simulink library "twolinkslib"  (R2019a)
settings: Solver=VariableStepAuto  StartTime=0.0  StopTime=10.0  RelTol=1e-3
libraries: $bdroot x5
settings Model: Creator=ah501846  LastModifiedBy=ah501846

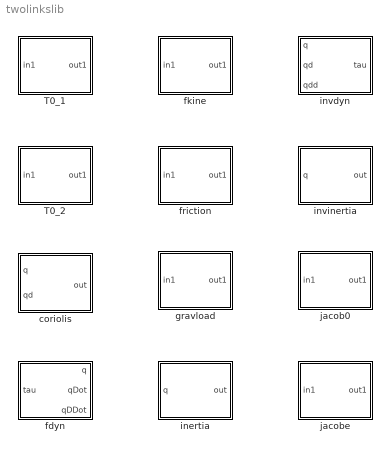
== system twolinkslib ==
  T0_1 : MATLAB Function  TreatAsAtomicUnit=on
  T0_2 : MATLAB Function  TreatAsAtomicUnit=on
  coriolis : Subsystem
  fdyn : Subsystem
  fkine : MATLAB Function  TreatAsAtomicUnit=on
  friction : MATLAB Function  TreatAsAtomicUnit=on
  gravload : MATLAB Function  TreatAsAtomicUnit=on
  inertia : Subsystem
  invdyn : Subsystem
  invinertia : Subsystem
  jacob0 : MATLAB Function  TreatAsAtomicUnit=on
  jacobe : MATLAB Function  TreatAsAtomicUnit=on

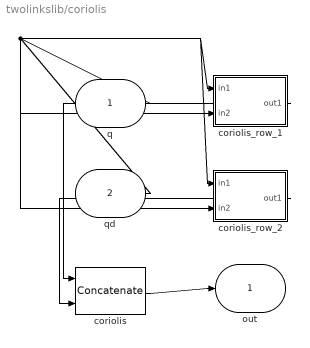
== system twolinkslib/coriolis ==
  q : Inport
  qd : Inport  Port=2
  coriolis : Concatenate  Mode=Multidimensional array
  coriolis_row_1 : MATLAB Function  TreatAsAtomicUnit=on
  coriolis_row_2 : MATLAB Function  TreatAsAtomicUnit=on
  out : Outport
  wires:
  coriolis/1 -> out/1
  coriolis_row_1/1(out1) -> coriolis/1
  q/1 -> coriolis_row_1/1(in1), coriolis_row_2/1(in1)
  qd/1 -> coriolis_row_1/2(in2), coriolis_row_2/2(in2)
  coriolis_row_2/1(out1) -> coriolis/2

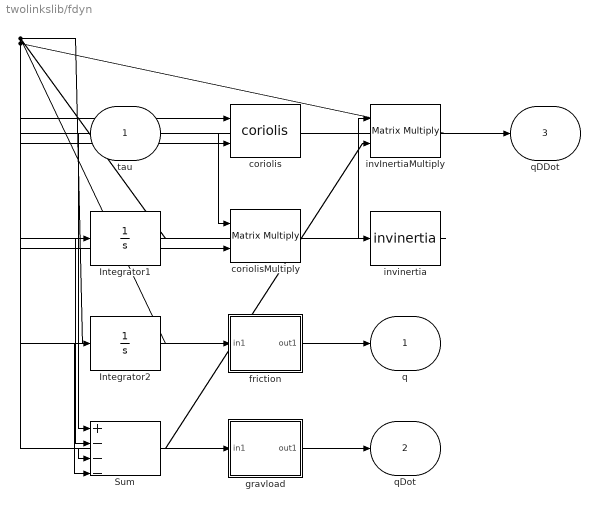
== system twolinkslib/fdyn ==
  tau : Inport
  Integrator1 : Integrator
  Integrator2 : Integrator
  Sum : Sum  Inputs=|+---  SaturateOnIntegerOverflow=on  InputSameDT=on  OutDataTypeStr=Inherit: Same as first input
  coriolis : $bdroot/coriolis  SystemSampleTime=-1
  coriolisMultiply : Product  Multiplication=Matrix(*)  SaturateOnIntegerOverflow=on  RndMeth=Zero  InputSameDT=on  OutDataTypeStr=Inherit: Same as first input
  friction : MATLAB Function  TreatAsAtomicUnit=on
  gravload : MATLAB Function  TreatAsAtomicUnit=on
  invInertiaMultiply : Product  Multiplication=Matrix(*)  SaturateOnIntegerOverflow=on  RndMeth=Zero  InputSameDT=on  OutDataTypeStr=Inherit: Same as first input
  invinertia : $bdroot/invinertia  SystemSampleTime=-1
  q : Outport
  qDot : Outport  Port=2
  qDDot : Outport  Port=3
  wires:
  tau/1 -> Sum/1
  invInertiaMultiply/1 -> qDDot/1, Integrator1/1
  Integrator1/1 -> Integrator2/1, qDot/1, coriolis/2, coriolisMultiply/2, friction/1(in1)
  Integrator2/1 -> q/1, coriolis/1, gravload/1(in1), invinertia/1
  invinertia/1 -> invInertiaMultiply/1
  Sum/1 -> invInertiaMultiply/2
  coriolisMultiply/1 -> Sum/2
  gravload/1(out1) -> Sum/3
  friction/1(out1) -> Sum/4
  coriolis/1 -> coriolisMultiply/1

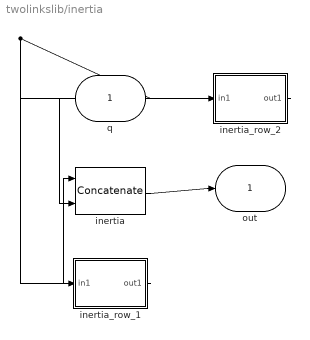
== system twolinkslib/inertia ==
  q : Inport
  inertia : Concatenate  Mode=Multidimensional array
  inertia_row_1 : MATLAB Function  TreatAsAtomicUnit=on
  inertia_row_2 : MATLAB Function  TreatAsAtomicUnit=on
  out : Outport
  wires:
  inertia/1 -> out/1
  inertia_row_1/1(out1) -> inertia/1
  q/1 -> inertia_row_1/1(in1), inertia_row_2/1(in1)
  inertia_row_2/1(out1) -> inertia/2

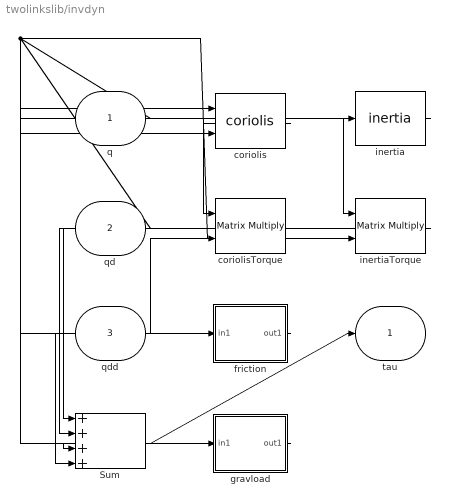
== system twolinkslib/invdyn ==
  q : Inport
  qd : Inport  Port=2
  qdd : Inport  Port=3
  Sum : Sum  Inputs=++++  SaturateOnIntegerOverflow=on  InputSameDT=on  OutDataTypeStr=Inherit: Same as first input
  coriolis : $bdroot/coriolis  SystemSampleTime=-1
  coriolisTorque : Product  Multiplication=Matrix(*)  SaturateOnIntegerOverflow=on  RndMeth=Zero  InputSameDT=on  OutDataTypeStr=Inherit: Same as first input
  friction : MATLAB Function  TreatAsAtomicUnit=on
  gravload : MATLAB Function  TreatAsAtomicUnit=on
  inertia : $bdroot/inertia  SystemSampleTime=-1
  inertiaTorque : Product  Multiplication=Matrix(*)  SaturateOnIntegerOverflow=on  RndMeth=Zero  InputSameDT=on  OutDataTypeStr=Inherit: Same as first input
  tau : Outport
  wires:
  q/1 -> inertia/1, coriolis/1, gravload/1(in1)
  qd/1 -> coriolis/2, friction/1(in1), coriolisTorque/2
  inertia/1 -> inertiaTorque/1
  qdd/1 -> inertiaTorque/2
  coriolis/1 -> coriolisTorque/1
  inertiaTorque/1 -> Sum/1
  coriolisTorque/1 -> Sum/2
  gravload/1(out1) -> Sum/3
  friction/1(out1) -> Sum/4
  Sum/1 -> tau/1

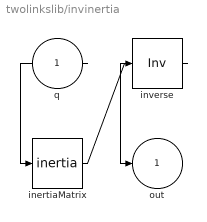
== system twolinkslib/invinertia ==
  q : Inport
  inertiaMatrix : $bdroot/inertia  SystemSampleTime=-1
  inverse : Product  Inputs=/  Multiplication=Matrix(*)
  out : Outport
  wires:
  q/1 -> inertiaMatrix/1
  inertiaMatrix/1 -> inverse/1
  inverse/1 -> out/1

== matlab function twolinkslib/inertia/inertia_row_2 ==
  data: in1 input; out1 output
function out1 = inertia_row_2(in1)
%#codegen

%    This function was generated by the Symbolic Math Toolbox version 8.3.
%    26-Apr-2019 09:45:12

q2 = in1(:,2);
out1 = [cos(q2)./2.0+1.0./4.0,1.0./4.0];

== matlab function twolinkslib/inertia/inertia_row_1 ==
  data: in1 input; out1 output
function out1 = inertia_row_1(in1)
%#codegen

%    This function was generated by the Symbolic Math Toolbox version 8.3.
%    26-Apr-2019 09:45:12

q2 = in1(:,2);
t2 = cos(q2);
out1 = [t2+3.0./2.0,t2./2.0+1.0./4.0];

== matlab function twolinkslib/fkine ==
  data: in1 input; out1 output
function out1 = fkine(in1)
%#codegen

%    This function was generated by the Symbolic Math Toolbox version 8.3.
%    26-Apr-2019 09:45:03

q1 = in1(:,1);
q2 = in1(:,2);
t2 = q1+q2;
t3 = cos(t2);
t4 = sin(t2);
out1 = reshape([t3,0.0,t4,0.0,-t4,0.0,t3,0.0,0.0,-1.0,0.0,0.0,t3+cos(q1),0.0,t4+sin(q1),1.0],[4,4]);

== matlab function twolinkslib/T0_1 ==
  data: in1 input; out1 output
function out1 = T0_1(in1)
%#codegen

%    This function was generated by the Symbolic Math Toolbox version 8.3.
%    26-Apr-2019 09:45:03

q1 = in1(:,1);
t2 = cos(q1);
t3 = sin(q1);
out1 = reshape([t2,0.0,t3,0.0,-t3,0.0,t2,0.0,0.0,-1.0,0.0,0.0,t2,0.0,t3,1.0],[4,4]);

== matlab function twolinkslib/T0_2 ==
  data: in1 input; out1 output
function out1 = T0_2(in1)
%#codegen

%    This function was generated by the Symbolic Math Toolbox version 8.3.
%    26-Apr-2019 09:45:04

q1 = in1(:,1);
q2 = in1(:,2);
t2 = cos(q1);
t3 = cos(q2);
t4 = sin(q1);
t5 = sin(q2);
t6 = t2.*t3;
t7 = t2.*t5;
t8 = t3.*t4;
t9 = t4.*t5;
t10 = -t9;
t11 = t6+t10;
out1 = reshape([t11,0.0,t7+t8,0.0,-t7-t8,0.0,t11,0.0,0.0,-1.0,0.0,0.0,t2+t11,0.0,t4+t7+t8,1.0],[4,4]);

== matlab function twolinkslib/jacob0 ==
  data: in1 input; out1 output
function out1 = jacob0(in1)
%#codegen

%    This function was generated by the Symbolic Math Toolbox version 8.3.
%    26-Apr-2019 09:45:06

q1 = in1(:,1);
q2 = in1(:,2);
t2 = cos(q2);
t3 = sin(q2);
t4 = q1+q2;
t5 = t2+1.0;
t6 = cos(t4);
t7 = sin(t4);
out1 = reshape([t3.*t6-t5.*t7,0.0,t3.*t7+t5.*t6,0.0,-1.0,0.0,-t7,0.0,t6,0.0,-1.0,0.0],[6,2]);

== matlab function twolinkslib/jacobe ==
  data: in1 input; out1 output
function out1 = jacobe(in1)
%#codegen

%    This function was generated by the Symbolic Math Toolbox version 8.3.
%    26-Apr-2019 09:45:07

q2 = in1(:,2);
out1 = reshape([sin(q2),cos(q2)+1.0,0.0,0.0,0.0,1.0,0.0,1.0,0.0,0.0,0.0,1.0],[6,2]);

== matlab function twolinkslib/gravload ==
  data: in1 input; out1 output
function out1 = gravload(in1)
%#codegen

%    This function was generated by the Symbolic Math Toolbox version 8.3.
%    26-Apr-2019 09:45:09

q1 = in1(:,1);
q2 = in1(:,2);
t2 = q1+q2;
t3 = cos(t2);
t4 = t3.*(9.81e+2./2.0e+2);
out1 = [t4+cos(q1).*1.4715e+1,t4];

== matlab function twolinkslib/coriolis/coriolis_row_1 ==
  data: in1 input; out1 output; in2 input
function out1 = coriolis_row_1(in1,in2)
%#codegen

%    This function was generated by the Symbolic Math Toolbox version 8.3.
%    26-Apr-2019 09:45:16

q2 = in1(:,2);
qd1 = in2(:,1);
qd2 = in2(:,2);
t2 = sin(q2);
out1 = [qd2.*t2.*(-1.0./2.0),t2.*(qd1+qd2).*(-1.0./2.0)];

== matlab function twolinkslib/coriolis/coriolis_row_2 ==
  data: in1 input; out1 output; in2 input
function out1 = coriolis_row_2(in1,in2)
%#codegen

%    This function was generated by the Symbolic Math Toolbox version 8.3.
%    26-Apr-2019 09:45:16

q2 = in1(:,2);
qd1 = in2(:,1);
out1 = [(qd1.*sin(q2))./2.0,0.0];

== matlab function twolinkslib/friction ==
  data: in1 input; out1 output
function out1 = friction(in1)
%#codegen

%    This function was generated by the Symbolic Math Toolbox version 8.3.
%    26-Apr-2019 09:45:18

out1 = [0.0,0.0];

== matlab function twolinkslib/fdyn/gravload ==
  data: in1 input; out1 output
function out1 = gravload(in1)
%#codegen

%    This function was generated by the Symbolic Math Toolbox version 8.3.
%    26-Apr-2019 09:45:09

q1 = in1(:,1);
q2 = in1(:,2);
t2 = q1+q2;
t3 = cos(t2);
t4 = t3.*(9.81e+2./2.0e+2);
out1 = [t4+cos(q1).*1.4715e+1,t4];

== matlab function twolinkslib/fdyn/friction ==
  data: in1 input; out1 output
function out1 = friction(in1)
%#codegen

%    This function was generated by the Symbolic Math Toolbox version 8.3.
%    26-Apr-2019 09:45:18

out1 = [0.0,0.0];

== matlab function twolinkslib/invdyn/gravload ==
  data: in1 input; out1 output
function out1 = gravload(in1)
%#codegen

%    This function was generated by the Symbolic Math Toolbox version 8.3.
%    26-Apr-2019 09:45:09

q1 = in1(:,1);
q2 = in1(:,2);
t2 = q1+q2;
t3 = cos(t2);
t4 = t3.*(9.81e+2./2.0e+2);
out1 = [t4+cos(q1).*1.4715e+1,t4];

== matlab function twolinkslib/invdyn/friction ==
  data: in1 input; out1 output
function out1 = friction(in1)
%#codegen

%    This function was generated by the Symbolic Math Toolbox version 8.3.
%    26-Apr-2019 09:45:18

out1 = [0.0,0.0];
